simulink model "Main_simulation_optimised_accel_testbed"  (R2017b)
settings: Solver=FixedStepDiscrete  StartTime=0  StopTime=2474  RelTol=1e-3  EnableMultiTasking=on
PreLoadFcn:
  | Ts=2e-6;
undefined symbols (not defined in the file): Batt, BatteryCback, BatteryLoadFcn, DiscIntNeverNeededParam, Discrete, gcbh, Ion, Lithium, sigbuilder_block, sps_rtmsupport, spsBatteryModel
libraries: powerlib x53, electricdrivelib x6, simulink x6, autolibshared x6, powerlib_meascontrol x4, sdolib x3, spsDrivesDcBusModel x1, spsDrivesPrivateModels x1, spsDrivesOutputSelector x1, spsDrivesSpeedControllerModel x1
(part 3 of 3)

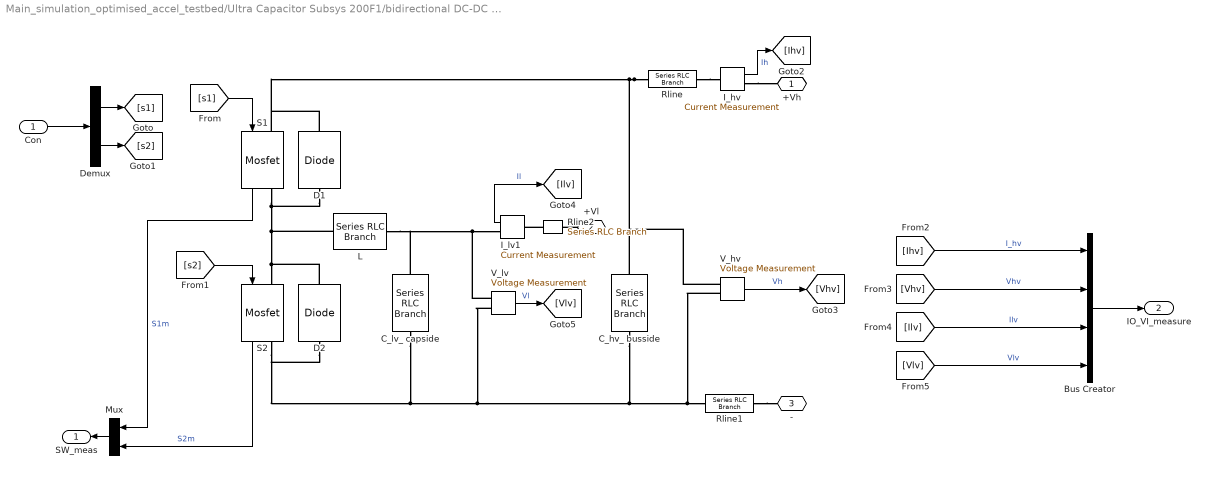
== system Main_simulation_optimised_accel_testbed/Ultra Capacitor Subsys 200F1/bidirectional DC-DC converter ==
  Con : Inport
  Bus Creator : BusCreator  Inputs=4
  C_hv_ busside : powerlib/Elements/Series RLC Branch  LConnTagsString=__new0  RConnTagsString=__new0  BranchType=RC  Resistance=0.09  Inductance=220e-6  SetiL0=off  InitialCurrent=0  Capacitance=447e-6  Setx0=off  InitialVoltage=0  Measurements=None
  C_lv_ capside : powerlib/Elements/Series RLC Branch  LConnTagsString=__new0  RConnTagsString=__new0  BranchType=RC  Resistance=0.08  Inductance=220e-6  SetiL0=off  InitialCurrent=0  Capacitance=447e-6  Setx0=off  InitialVoltage=0  Measurements=None
  D1 : powerlib/Power Electronics/Diode  Ron=0.001  Lon=0  Vf=0.8  IC=0  UseSnubber=0  Rs=inf  Cs=250e-9  Measurements=off
  D2 : powerlib/Power Electronics/Diode  Ron=0.001  Lon=0  Vf=0.8  IC=0  UseSnubber=0  Rs=inf  Cs=250e-9  Measurements=off
  Demux : Demux  Outputs=2
  I_hv : powerlib/Measurements/Current Measurement  PhasorSimulation=off  OutputType=Complex  PSBequivalent=0
  I_lv1 : powerlib/Measurements/Current Measurement  PhasorSimulation=off  OutputType=Complex  PSBequivalent=0
  L : powerlib/Elements/Series RLC Branch  LConnTagsString=__new0  RConnTagsString=__new0  BranchType=RL  Resistance=0.05  Inductance=100e-6  SetiL0=off  InitialCurrent=0  Capacitance=1e-6  Setx0=off  InitialVoltage=0  Measurements=None
  Mux : Mux  Inputs=2
  Rline : powerlib/Elements/Series RLC Branch  LConnTagsString=__new0  RConnTagsString=__new0  BranchType=R  Resistance=0.08  Inductance=220e-6  SetiL0=off  InitialCurrent=0  Capacitance=447e-6  Setx0=off  InitialVoltage=0  Measurements=None
  Rline1 : powerlib/Elements/Series RLC Branch  LConnTagsString=__new0  RConnTagsString=__new0  BranchType=R  Resistance=0.08  Inductance=220e-6  SetiL0=off  InitialCurrent=0  Capacitance=447e-6  Setx0=off  InitialVoltage=0  Measurements=None
  Rline2 : powerlib/Elements/Series RLC Branch  LConnTagsString=__new0  RConnTagsString=__new0  BranchType=R  Resistance=0.08  Inductance=220e-6  SetiL0=off  InitialCurrent=0  Capacitance=447e-6  Setx0=off  InitialVoltage=0  Measurements=None
  S1 : powerlib/Power Electronics/Mosfet  Ron=0.1  Lon=0  Rd=0.01  Vfd=0  IC=0  Rs=1e5  Cs=inf  Measurements=on
  S2 : powerlib/Power Electronics/Mosfet  Ron=0.1  Lon=0  Rd=0.01  Vfd=0  IC=0  Rs=1e5  Cs=inf  Measurements=on
  V_hv : powerlib/Measurements/Voltage Measurement  PhasorSimulation=off  OutputType=Complex  PSBequivalent=0
  V_lv : powerlib/Measurements/Voltage Measurement  PhasorSimulation=off  OutputType=Complex  PSBequivalent=0
  +Vh : PMIOPort  Port=1  Side=Left
  +Vl : PMIOPort  Port=2  Side=Right
  - : PMIOPort  Port=3  Side=Right
  SW_meas : Outport
  IO_VI_measure : Outport  Port=2
  wires:
  Mux/1 -> SW_meas/1
  [s1] -> S1/1
  [s2] -> S2/1
  Demux/2 -> [s2]
  Demux/1 -> [s1]
  Con/1 -> Demux/1
  S1/1 -> Mux/1  "S1m"
  S2/1 -> Mux/2  "S2m"
  I_hv/1 -> [Ihv]  "Ih"
  V_hv/1 -> [Vhv]  "Vh"
  I_lv1/1 -> [Ilv]  "Il"
  V_lv/1 -> [Vlv]  "Vl"
  [Ihv] -> Bus Creator/1  "I_hv"
  [Vhv] -> Bus Creator/2  "Vhv"
  [Ilv] -> Bus Creator/3  "Ilv"
  [Vlv] -> Bus Creator/4  "Vlv"
  Bus Creator/1 -> IO_VI_measure/1
  connections:
  L/RConn1 -- C_lv_ capside/LConn1 -- I_lv1/RConn1 -- V_lv/LConn1
  C_lv_ capside/RConn1 -- S2/RConn1 -- D2/LConn1 -- V_lv/LConn2 -- C_hv_ busside/RConn1 -- V_hv/LConn2 -- Rline1/RConn1
  Rline/RConn1 -- V_hv/LConn1 -- C_hv_ busside/LConn1 -- S1/LConn1 -- D1/RConn1
  S1/RConn1 -- D1/LConn1 -- D2/RConn1 -- S2/LConn1 -- L/LConn1
  +Vl/RConn1 -- Rline2/LConn1
  I_hv/RConn1 -- +Vh/RConn1
  Rline/LConn1 -- I_hv/LConn1
  Rline1/LConn1 -- -/RConn1
  Rline2/RConn1 -- I_lv1/LConn1

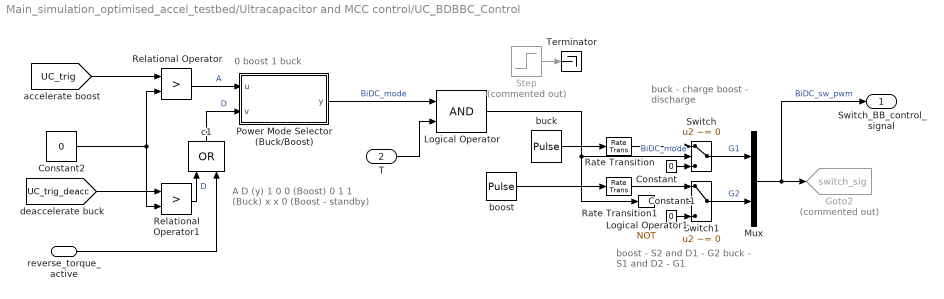
== system Main_simulation_optimised_accel_testbed/Ultracapacitor and MCC control/UC_BDBBC_Control ==
  note: A	D	(y)
      | 1	0	0 (Boost)
      | 0	1	1 (Buck)
      | x	x	0 (Boost - standby)
  note: buck - charge
      | boost - discharge
  note: 0 boost 1 buck
  note: boost - S2 and D1 - G2
      | buck - S1 and D2 - G1
  reverse_torque_active : Inport
  T : Inport  Port=2
  Constant : Constant  Value=0
  Constant1 : Constant  Value=0
  Constant2 : Constant  Value=0
  Goto2 : Goto  Commented=on  GotoTag=switch_sig  TagVisibility=global
  Logical Operator : Logic  IconShape=distinctive  AllPortsSameDT=off  OutDataTypeStr=boolean
  Logical Operator1 : Logic  Operator=NOT  IconShape=distinctive  AllPortsSameDT=off  OutDataTypeStr=boolean
  Mux : Mux  Inputs=2
  Power Mode Selector (Buck/Boost) : MATLAB Function  TreatAsAtomicUnit=on
  Rate Transition : RateTransition
  Rate Transition1 : RateTransition
  Relational Operator : RelationalOperator  Operator=>  OutDataTypeStr=boolean  RndMeth=Simplest
  Relational Operator1 : RelationalOperator  Operator=>  OutDataTypeStr=boolean  RndMeth=Simplest
  Step : Step  Commented=on  Time=5  SampleTime=0
  Switch : Switch  Criteria=u2 ~= 0
  Switch1 : Switch  Criteria=u2 ~= 0
  Terminator : Terminator
  boost : DiscretePulseGenerator  PulseType=Time based  Period=1/10e3  PulseWidth=85
  buck : DiscretePulseGenerator  PulseType=Time based  Period=1/10e3  PulseWidth=20
  c1 : Logic  Operator=OR  AllPortsSameDT=off  OutDataTypeStr=boolean
  Switch_BB_control_signal : Outport
  wires:
  Switch1/1 -> Mux/2  "G2"
  Logical Operator1/1 -> Switch1/2
  Mux/1 -> Switch_BB_control_signal/1, Goto2/1  "BiDC_sw_pwm"
  buck/1 -> Rate Transition/1
  boost/1 -> Rate Transition1/1
  Switch/1 -> Mux/1  "G1"
  Constant/1 -> Switch/3
  Constant1/1 -> Switch1/3
  Step/1 -> Terminator/1
  Logical Operator/1 -> Logical Operator1/1, Switch/2  "BiDC_mode"
  [UC_trig] -> Relational Operator/1
  Constant2/1 -> Relational Operator/2, Relational Operator1/2
  Relational Operator/1 -> Power Mode Selector (Buck/Boost)/1(u)  "A"
  c1/1 -> Power Mode Selector (Buck/Boost)/2(v)  "D"
  Rate Transition/1 -> Switch/1
  Rate Transition1/1 -> Switch1/1
  reverse_torque_active/1 -> c1/2
  [UC_trig_deacc] -> Relational Operator1/1
  Relational Operator1/1 -> c1/1  "D"
  Power Mode Selector (Buck/Boost)/1(y) -> Logical Operator/1  "BiDC_mode"
  T/1 -> Logical Operator/2

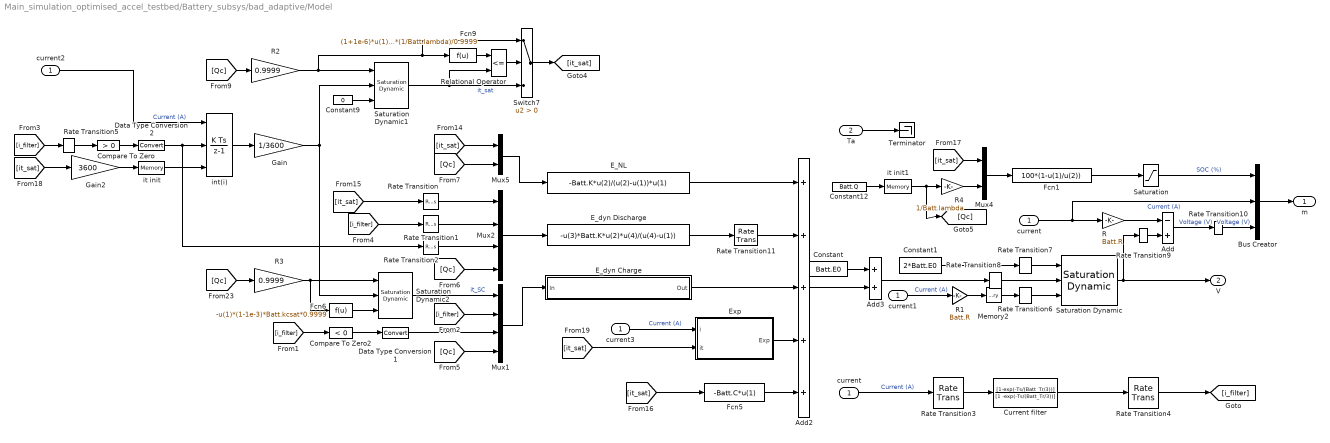
== system Main_simulation_optimised_accel_testbed/Battery_subsys/bad_adaptive/Model ==
  current : Inport
  Ta : Inport  Port=2
  Add : Sum  Inputs=-+
  Add2 : Sum  Inputs=+++++
  Add3 : Sum
  Bus Creator : BusCreator  Inputs=3
  Compare To Zero : simulink/Logic and Bit Operations/Compare To Zero  relop=>  OutDataTypeStr=uint8
  Compare To Zero2 : simulink/Logic and Bit Operations/Compare To Zero  relop=<  OutDataTypeStr=uint8
  Constant : Constant  Value=Batt.E0
  Constant1 : Constant  Value=2*Batt.E0
  Constant12 : Constant  Value=Batt.Q
  Constant9 : Constant  Value=0
  Current filter : DiscreteTransferFcn  Numerator=[1-exp(-Ts/(Batt_Tr/3))]  Denominator=[1 -exp(-Ts/(Batt_Tr/3))]  SampleTime=Ts
  Data Type Conversion1 : DataTypeConversion
  Data Type Conversion2 : DataTypeConversion
  E_NL : Fcn  Expr=-Batt.K*u(2)/(u(2)-u(1))*u(1)
  E_dyn Charge : Subsystem
  E_dyn Discharge : Fcn  Expr=-u(3)*Batt.K*u(2)*u(4)/(u(4)-u(1))
  Exp : Subsystem
  Fcn1 : Fcn  Expr=100*(1-u(1)/u(2))
  Fcn5 : Fcn  Expr=-Batt.C*u(1)
  Fcn6 : Fcn  Expr=-u(1)*(1-1e-3)*Batt.kcsat*0.9999
  Fcn9 : Fcn  Expr=(1+1e-6)*u(1)*(1/Batt.lambda)/0.9999
  Gain : Gain  Gain=1/3600
  Gain2 : Gain  Gain=3600
  Memory2 : Memory  InheritSampleTime=on
  Mux1 : Mux
  Mux2 : Mux
  Mux4 : Mux  Inputs=2
  Mux5 : Mux  Inputs=2
  R : Gain  Gain=Batt.R
  R1 : Gain  Gain=Batt.R
  R2 : Gain  Gain=0.9999
  R3 : Gain  Gain=0.9999
  R4 : Gain  Gain=1/Batt.lambda
  Rate Transition{,1..11} (12 alike) : RateTransition
  Relational Operator : RelationalOperator  Operator=<=  RndMeth=Simplest
  Saturation : Saturate  UpperLimit=100  LowerLimit=0
  Saturation Dynamic : simulink/Discontinuities/Saturation Dynamic  OutMin=[]  OutMax=[]  OutDataTypeStr=Inherit: Same as second input  OutDataType=sfix(16)  OutScaling=2^-10  DoSatur=off
  Saturation Dynamic1 : simulink/Discontinuities/Saturation Dynamic  OutMin=[]  OutMax=[]  OutDataTypeStr=Inherit: Same as second input  OutDataType=sfix(16)  OutScaling=2^-10  DoSatur=off
  Saturation Dynamic2 : simulink/Discontinuities/Saturation Dynamic  OutMin=[]  OutMax=[]  OutDataTypeStr=Inherit: Same as second input  OutDataType=sfix(16)  OutScaling=2^-10  DoSatur=off
  Switch7 : Switch  Criteria=u2 > Threshold
  Terminator : Terminator
  "current " : InportShadow
  current1 : InportShadow
  current2 : InportShadow
  current3 : InportShadow
  int(i) : DiscreteIntegrator  ExternalReset=rising  InitialConditionSource=external  SampleTime=Ts  LimitOutput=on  UpperSaturationLimit=Batt.Qmax*3600  ICPrevOutput=DiscIntNeverNeededParam  ICPrevScaledInput=DiscIntNeverNeededParam
  it init : Memory  InitialCondition=(1-SOC/100)*Batt.Q*(1/Batt.lambda)*3600
  it init1 : Memory  InitialCondition=Batt.Q
  m : Outport
  V : Outport  Port=2
  wires:
  Rate Transition11/1 -> Add2/2
  Rate Transition10/1 -> Bus Creator/3  "Voltage (V)"
  Rate Transition9/1 -> Add/2
  Rate Transition8/1 -> Saturation Dynamic/2
  Rate Transition7/1 -> Saturation Dynamic/1
  Rate Transition6/1 -> Saturation Dynamic/3
  Rate Transition5/1 -> Compare To Zero/1
  Rate Transition4/1 -> [i_filter]
  Rate Transition3/1 -> Current filter/1
  Rate Transition2/1 -> Mux2/3
  Rate Transition1/1 -> Mux2/2
  Rate Transition/1 -> Mux2/1
  Mux2/1 -> E_dyn Discharge/1
  E_dyn Discharge/1 -> Rate Transition11/1
  current/1 -> R/1, Bus Creator/2  "Current (A)"
  int(i)/1 -> Gain/1
  Fcn1/1 -> Saturation/1
  Add/1 -> Rate Transition10/1  "Voltage (V)"
  R/1 -> Add/1
  Bus Creator/1 -> m/1
  Constant/1 -> Add3/1
  Mux1/1 -> E_dyn Charge/1(In)
  it init/1 -> int(i)/3
  Compare To Zero/1 -> Data Type Conversion2/1
  Compare To Zero2/1 -> Data Type Conversion1/1
  Data Type Conversion2/1 -> int(i)/2, Rate Transition2/1
  Gain2/1 -> it init/1
  Exp/1(Exp) -> Add2/4
  Data Type Conversion1/1 -> Mux1/3
  Saturation Dynamic2/1 -> Mux1/1  "it_SC"
  Constant1/1 -> Rate Transition7/1
  Add3/1 -> Rate Transition8/1
  E_NL/1 -> Add2/1
  E_dyn Charge/1(Out) -> Add2/3
  Fcn5/1 -> Add2/5
  Mux4/1 -> Fcn1/1
  Mux5/1 -> E_NL/1
  Fcn6/1 -> Saturation Dynamic2/3
  current2/1 -> int(i)/1  "Current (A)"
  current3/1 -> Exp/1(i)  "Current (A)"
  "current "/1 -> Rate Transition3/1  "Current (A)"
  Current filter/1 -> Rate Transition4/1
  [i_filter] -> Compare To Zero2/1
  [i_filter] -> Mux1/2
  [i_filter] -> Rate Transition5/1
  [i_filter] -> Rate Transition1/1
  [Qc] -> Mux1/4
  [Qc] -> Mux2/4
  it init1/1 -> [Qc], R4/1
  [Qc] -> R2/1
  [it_sat] -> Mux5/1
  [it_sat] -> Rate Transition/1
  [it_sat] -> Fcn5/1
  [it_sat] -> Mux4/1
  [it_sat] -> Gain2/1
  [it_sat] -> Exp/2(it)
  [Qc] -> R3/1
  R3/1 -> Fcn6/1, Saturation Dynamic2/1
  Add2/1 -> Add3/2
  R4/1 -> Mux4/2
  Saturation/1 -> Bus Creator/1  "SOC (%)"
  Saturation Dynamic/1 -> Rate Transition9/1, V/1
  [Qc] -> Mux5/2
  Gain/1 -> Saturation Dynamic1/2, Saturation Dynamic2/2
  Constant9/1 -> Saturation Dynamic1/3
  current1/1 -> R1/1  "Current (A)"
  Memory2/1 -> Rate Transition6/1
  R1/1 -> Memory2/1
  Saturation Dynamic1/1 -> Relational Operator/2, Switch7/3  "it_sat"
  R2/1 -> Switch7/1, Fcn9/1, Saturation Dynamic1/1
  Switch7/1 -> [it_sat]
  Fcn9/1 -> Relational Operator/1
  Relational Operator/1 -> Switch7/2
  Ta/1 -> Terminator/1
  Constant12/1 -> it init1/1

== system Main_simulation_optimised_accel_testbed/PMSM Drive vehicle/PM Synchronous Motor Drive/Measures ==
  Current Measurement : powerlib/Measurements/Current Measurement  Tag=PoWeRsYsTeMmEaSuReMeNt  PhasorSimulation=off  OutputType=Magnitude  PSBequivalent=0
  Current Measurement1 : powerlib/Measurements/Current Measurement  Tag=PoWeRsYsTeMmEaSuReMeNt  PhasorSimulation=off  OutputType=Magnitude  PSBequivalent=0
  Current Measurement2 : powerlib/Measurements/Current Measurement  Tag=PoWeRsYsTeMmEaSuReMeNt  PhasorSimulation=off  OutputType=Magnitude  PSBequivalent=0
  Mux1 : Mux  Inputs=3
  Ta : PMIOPort  Port=1  Side=Left
  Tb : PMIOPort  Port=2  Side=Left
  Tc : PMIOPort  Port=3  Side=Left
  Mta : PMIOPort  Port=4  Side=Right
  Mtb : PMIOPort  Port=5  Side=Right
  Mtc : PMIOPort  Port=6  Side=Right
  I_abc : Outport
  wires:
  Current Measurement1/1 -> Mux1/2
  Current Measurement/1 -> Mux1/1
  Current Measurement2/1 -> Mux1/3
  Mux1/1 -> I_abc/1
  connections:
  Current Measurement1/RConn1 -- Mtb/RConn1
  Tb/RConn1 -- Current Measurement1/LConn1
  Current Measurement/RConn1 -- Mta/RConn1
  Ta/RConn1 -- Current Measurement/LConn1
  Tc/RConn1 -- Current Measurement2/LConn1
  Current Measurement2/RConn1 -- Mtc/RConn1

== system Main_simulation_optimised_accel_testbed/Battery_subsys/bad_adaptive/Model/E_dyn Charge ==
  In : Inport
  Charge Lead-Acid : Fcn  Expr=-u(3)*Batt.K*u(2)*(Batt.Q/(u(1)+Batt.Q*Batt.kc))
  Charge Li-Ion : Fcn  Expr=-u(3)*Batt.K*u(2)*u(4)/(u(1)+u(4)*Batt.kc)
  Charge NiCD : Fcn  Expr=-u(3)*Batt.K*u(2)*(Batt.Q/(abs(u(1))+Batt.Q*Batt.kc))
  Charge NiMH : Fcn  Expr=-u(3)*Batt.K*u(2)*(Batt.Q/(abs(u(1))+Batt.Q*Batt.kc))
  Constant : Constant  Value=BatType
  Constant1 : Constant  Value=BatType == 2  OutDataTypeStr=double
  Constant2 : Constant  Value=BatType == 4  OutDataTypeStr=double
  Constant3 : Constant  Value=BatType == 3  OutDataTypeStr=double
  Constant4 : Constant  Value=BatType == 1  OutDataTypeStr=double
  Multiport Switch1 : MultiPortSwitch  Inputs=4
  Product{,1..3} (4 alike) : Product  RndMeth=Zero
  Rate Transition1 : RateTransition
  Out : Outport
  wires:
  Rate Transition1/1 -> Out/1
  In/1 -> Product3/2, Product/2, Product1/2, Product2/2
  Multiport Switch1/1 -> Rate Transition1/1
  Charge Li-Ion/1 -> Multiport Switch1/3
  Charge NiMH/1 -> Multiport Switch1/5
  Charge NiCD/1 -> Multiport Switch1/4
  Charge Lead-Acid/1 -> Multiport Switch1/2
  Constant/1 -> Multiport Switch1/1
  Product/1 -> Charge Li-Ion/1
  Constant1/1 -> Product/1
  Product1/1 -> Charge NiMH/1
  Constant2/1 -> Product1/1
  Product2/1 -> Charge NiCD/1
  Constant3/1 -> Product2/1
  Product3/1 -> Charge Lead-Acid/1
  Constant4/1 -> Product3/1

== system Main_simulation_optimised_accel_testbed/Battery_subsys/bad_adaptive/Model/Exp ==
  i : Inport
  it : Inport  Port=2
  Abs : Abs
  Add3 : Sum  Inputs=+-
  Compare To Zero2 : simulink/Logic and Bit Operations/Compare To Zero  relop=<  OutDataTypeStr=uint8
  Constant : Constant  Value=BatType
  Data Type Conversion1 : DataTypeConversion
  Discrete-Time Integrator : DiscreteIntegrator  InitialCondition=Batt.A*exp(-Batt.B*(1-SOC/100)*Batt.Q)  SampleTime=Ts  ICPrevOutput=DiscIntNeverNeededParam  ICPrevScaledInput=DiscIntNeverNeededParam
  Divide : Product  Inputs=**
  Gain1 : Gain  Gain=Batt.B/3600
  Gain4 : Gain  Gain=Batt.A
  Li-Ion : Fcn  Expr=Batt.A*exp(-Batt.B*u(1))
  Multiport Switch1 : MultiPortSwitch  Inputs=4
  Saturation : Saturate  UpperLimit=Batt.Qmax*(1/Batt.lambda)  LowerLimit=-inf
  Exp : Outport
  wires:
  Discrete-Time Integrator/1 -> Multiport Switch1/2, Multiport Switch1/4, Add3/2, Multiport Switch1/5
  Gain4/1 -> Add3/1
  Divide/1 -> Gain1/1
  Abs/1 -> Divide/1
  Add3/1 -> Divide/2
  Gain1/1 -> Discrete-Time Integrator/1
  i/1 -> Abs/1, Compare To Zero2/1
  Constant/1 -> Multiport Switch1/1
  it/1 -> Saturation/1
  Li-Ion/1 -> Multiport Switch1/3
  Multiport Switch1/1 -> Exp/1
  Compare To Zero2/1 -> Data Type Conversion1/1
  Data Type Conversion1/1 -> Gain4/1
  Saturation/1 -> Li-Ion/1

== matlab function Main_simulation_optimised_accel_testbed/Ultracapacitor and MCC control/UC_BDBBC_Control/Power Mode Selector (Buck//Boost) ==
  data: u input; y output; v input
function y = pmodeselect(u,v)

% U - accelerate
% V - decelerate

if u>0 && v<1   %accelerating
    y=0; % boost
elseif u<1 && v>0   %decelerating
    y=1; % buck
else    %default
    y=0; % default boost or standby for power dump
end
